simulink model "identifyOnHW"  (R2018b)
settings: Solver=FixedStepDiscrete  StartTime=0.0  StopTime=600  FixedStep=0.001  RelTol=1e-3
settings Model: Creator=Bondi  LastModifiedBy=Bondi

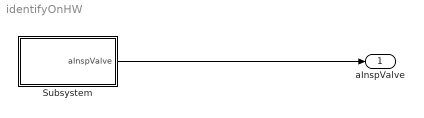
== system identifyOnHW ==
  Subsystem : Subsystem
  aInspValve : Outport  OutputWhenDisabled=reset  InitialOutput=0
  wires:
  Subsystem/1(aInspValve) -> aInspValve/1

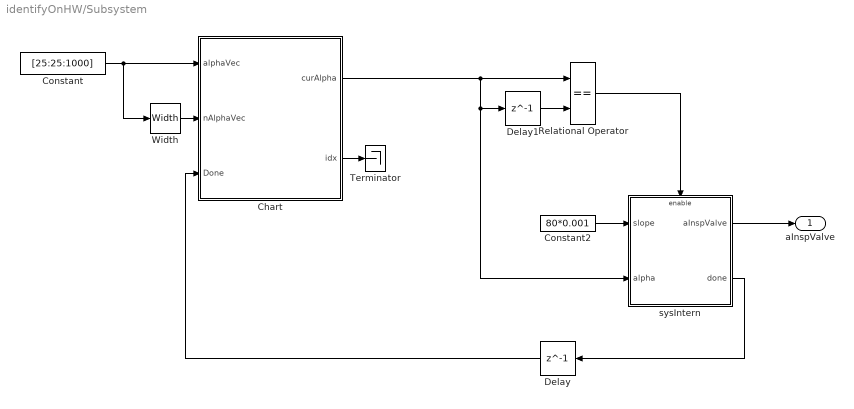
== system identifyOnHW/Subsystem ==
  Chart : Stateflow chart  TreatAsAtomicUnit=on
  Constant : Constant  Value=[25:25:1000]
  Constant2 : Constant  Value=80*0.001
  Delay : Delay  DelayLength=1  InitialCondition=false
  Delay1 : Delay  DelayLength=1
  Relational Operator : RelationalOperator  Operator===  OutDataTypeStr=boolean  RndMeth=Simplest
  Terminator : Terminator
  Width : Width
  sysIntern : Subsystem
  aInspValve : Outport  OutputWhenDisabled=reset  InitialOutput=0
  wires:
  Chart/1(curAlpha) -> sysIntern/2(alpha), Delay1/1, Relational Operator/1
  Constant/1 -> Width/1, Chart/1(alphaVec)
  sysIntern/1(aInspValve) -> aInspValve/1
  Width/1 -> Chart/2(nAlphaVec)
  Chart/2(idx) -> Terminator/1
  Relational Operator/1 -> sysIntern/Enable
  Constant2/1 -> sysIntern/1(slope)
  Delay/1 -> Chart/3(Done)
  sysIntern/2(done) -> Delay/1
  Delay1/1 -> Relational Operator/2

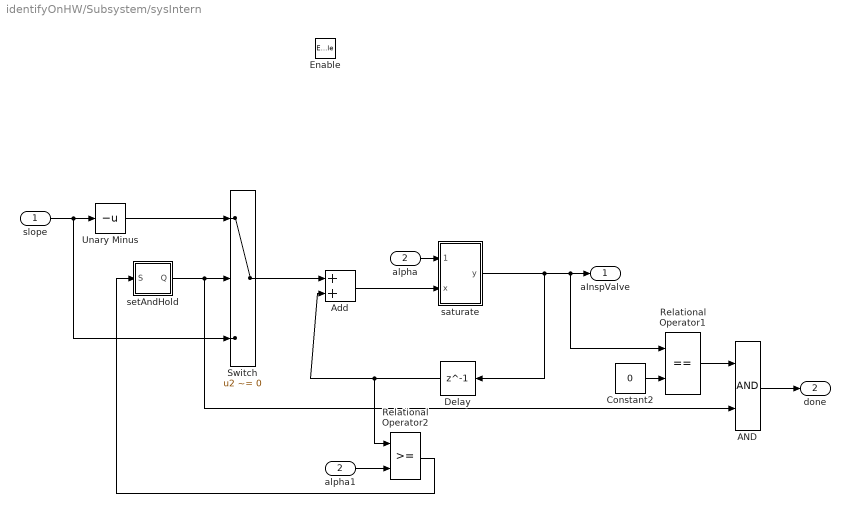
== system identifyOnHW/Subsystem/sysIntern ==
  slope : Inport
  alpha : Inport  Port=2
  Enable : EnablePort  StatesWhenEnabling=reset
  AND : Logic  AllPortsSameDT=off  OutDataTypeStr=boolean
  Add : Sum
  Constant2 : Constant  Value=0
  Delay : Delay  DelayLength=1
  Relational Operator1 : RelationalOperator  Operator===  OutDataTypeStr=boolean  RndMeth=Simplest
  Relational Operator2 : RelationalOperator  OutDataTypeStr=boolean  RndMeth=Simplest
  Switch : Switch  Criteria=u2 ~= 0
  Unary Minus : UnaryMinus
  alpha1 : InportShadow  Port=2
  saturate : Subsystem
  setAndHold : Subsystem
  aInspValve : Outport  OutputWhenDisabled=reset  InitialOutput=0
  done : Outport  Port=2  OutputWhenDisabled=reset  InitialOutput=false
  wires:
  Delay/1 -> Relational Operator2/1, Add/2
  Add/1 -> saturate/2(x)
  slope/1 -> Switch/3, Unary Minus/1
  Switch/1 -> Add/1
  Unary Minus/1 -> Switch/1
  Constant2/1 -> Relational Operator1/2
  AND/1 -> done/1
  saturate/1(y) -> Relational Operator1/1, aInspValve/1, Delay/1
  alpha/1 -> saturate/1(alpha)
  Relational Operator1/1 -> AND/1
  setAndHold/1(Q) -> AND/2, Switch/2
  Relational Operator2/1 -> setAndHold/1(S)
  alpha1/1 -> Relational Operator2/2

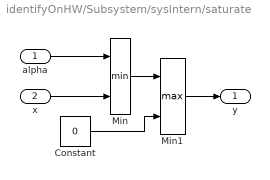
== system identifyOnHW/Subsystem/sysIntern/saturate ==
  alpha : Inport
  x : Inport  Port=2
  Constant : Constant  Value=0
  Min : MinMax  Inputs=2
  Min1 : MinMax  Function=max  Inputs=2
  y : Outport
  wires:
  Constant/1 -> Min1/2
  Min/1 -> Min1/1
  x/1 -> Min/2
  Min1/1 -> y/1
  alpha/1 -> Min/1

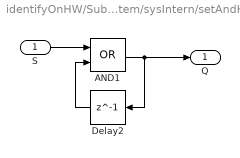
== system identifyOnHW/Subsystem/sysIntern/setAndHold ==
  S : Inport
  AND1 : Logic  Operator=OR  AllPortsSameDT=off  OutDataTypeStr=boolean
  Delay2 : Delay  DelayLength=1  InitialCondition=false
  Q : Outport  OutputWhenDisabled=reset  InitialOutput=0
  wires:
  Delay2/1 -> AND1/2
  S/1 -> AND1/1
  AND1/1 -> Q/1, Delay2/1

== stateflow chart identifyOnHW/Subsystem/Chart ==
  state y
  state RunAlphaValue
    en:
    curAlpha=alphaVec(idx)
  (junction 16) -> y [order 2]
  (junction 16) -> (junction 17) [order 1] : [idx<nAlphaVec]
  RunAlphaValue -> (junction 16) : [Done]
  (junction 17) -> RunAlphaValue : {idx=idx+1;}
  (default) -> RunAlphaValue : {idx=1;}
  data: alphaVec input; nAlphaVec input; curAlpha output; idx output; Done input
